simulink model "f28377S_DCDC_Buck"  (R2021b)
settings: Solver=FixedStepDiscrete  StartTime=0.0  StopTime=Inf  RelTol=1e-3  EnableMultiTasking=on
undefined symbols (not defined in the file or in its folder): GPTRIP1SEL, GPTRIP2SEL, TZ1, TZ2
libraries: c2837xDlib x3, c2802xlib x3, simulink x3, tiiqmathlib x2, c280xlib x2, c2000lib x1, demo_controls x1
settings Model: ExtModeTrigDuration=8  ExtModeTrigDurationFloating=10  ExtModeTrigDirection=either  ExtModeTrigLevel=0.500000  Creator=The MathWorks, Inc.  LastModifiedBy=The MathWorks, Inc.
settings SolverCC: AlgebraicLoopSolver=TrustRegion
settings DataIOCC: LimitDataPoints=on  SaveFormat=Array  SaveOutput=off  SaveTime=off  ReturnWorkspaceOutputs=off
settings OptimizationCC: DefaultParameterBehavior=Inlined  DefaultUnderspecifiedDataType=single  UseSpecifiedMinMax=on  InlineInvariantSignals=on  OptimizeBlockIOStorage=off  BufferReuse=off  GlobalBufferReuse=off  StrengthReduction=on  ExpressionFolding=off  PassReuseOutputArgsAs=Individual arguments  LocalBlockOutputs=off  NoFixptDivByZeroProtection=on  EfficientFloat2IntCast=on  LifeSpan=1  MaxStackSize=512  OptimizeDataStoreBuffers=off  BusAssignmentInplaceUpdate=off  EfficientTunableParamExpr=on
settings DebuggingCC: SolverPrmCheckMsg=warning  InheritedTsInSrcMsg=none  ParameterPrecisionLossMsg=none  SFUnexpectedBacktrackingDiag=warning  SFNoUnconditionalDefaultTransitionDiag=warning  SFExecutionAtInitializationDiag=none  SFMachineParentedDataDiag=warning  ArithmeticOperatorsInVariantConditions=warning
settings HardwareCC: ProdBitPerChar=16  ProdBitPerInt=16  ProdBitPerPointer=32  ProdBitPerSizeT=32  ProdBitPerPtrDiffT=32  ProdLargestAtomicInteger=Integer  ProdLargestAtomicFloat=None  ProdWordSize=16  ProdLongLongMode=on  ProdHWDeviceType=Texas Instruments->C2000
settings ModelReferenceCC: PropagateSignalLabelsOutOfModel=off
settings SFSimCC: SimUseLocalCustomCode=off  MATLABDynamicMemAlloc=off  CustomCodeUndefinedFunction=UseInterfaceOnly
settings RTWCC: Description=Embedded Coder  SystemTargetFile=ert.tlc  HardwareBoard=TI Delfino F2837xS  TemplateMakefile=ert_default_tmf  GenerateReport=on  RTWUseLocalCustomCode=off  Toolchain=Texas Instruments Code Composer Studio (C2000)  BuildConfiguration=Faster Runs  IncludeHyperlinkInReport=on  GenerateTraceInfo=on  GenerateTraceReport=on  GenerateTraceReportSl=on  GenerateTraceReportSf=on  GenerateTraceReportEml=on  GenerateCodeMetricsReport=on  GenerateCodeReplacementReport=on
settings CodeAppCC: IgnoreCustomStorageClasses=off  StateflowObjectComments=on
settings ERTTargetCC: CodeReplacementLibrary=TI C28x  UtilityFuncGeneration=Shared location  MultiwordLength=2048  IncludeMdlTerminateFcn=off  CombineSignalStateStructs=on  SupportAbsoluteTime=off  SupportNonFinite=off  SupportComplex=off  ExtModeMexFile=TIC2000ExternalModeOpen  ExtModeMexArgs=1 65 115385 30  ExtModeIntrfLevel=Level2 - Open  ERTFilePackagingFormat=Compact
settings ConfigComp: CovMetricSettings=dw  CovSaveCumulativeToWorkspaceVar=on  CovSaveSingleToWorkspaceVar=on  CovExternalEMLEnable=off  CovSFcnEnable=off
settings SimscapeCC: SimscapeNormalizeSystem=off
settings ConfigurationSet: Description=SimMechanics 2G

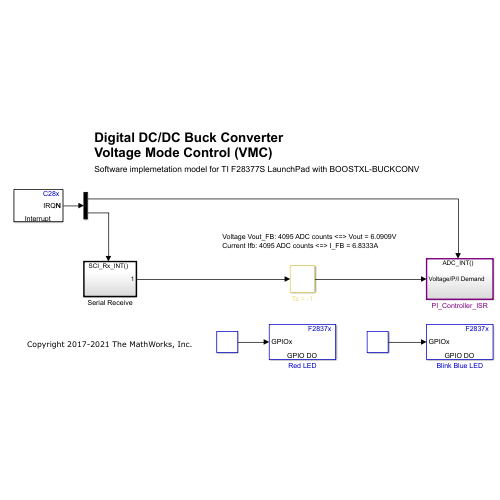
[thumbnail: Simulink's stored preview of the top-level diagram]
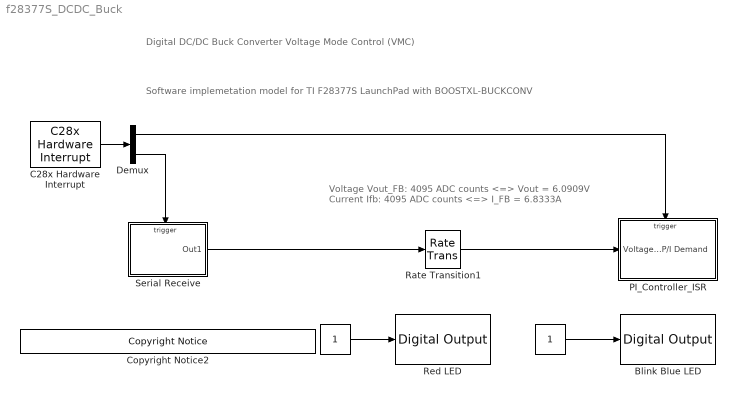
== system f28377S_DCDC_Buck ==
  note: Voltage Vout_FB: 4095 ADC counts <=> Vout = 6.0909V
      | Current Ifb: 4095 ADC counts <=> I_FB = 6.8333A
  note: Software implemetation model for TI F28377S LaunchPad with BOOSTXL-BUCKCONV
  note: Digital DC/DC Buck Converter
      | Voltage Mode Control (VMC)
  " " : Constant  OutDataTypeStr=uint16  SampleTime=0.5
  "   " : Constant  OutDataTypeStr=uint16  SampleTime=0.5
  Blink Blue LED : c2837xDlib/Digital Output  GPIO_Number=GPIO8~GPIO15  GPIO_Bit0=off  GPIO_BIT0_Toggle=off  GPIO_Bit1=off  GPIO_BIT1_Toggle=off  GPIO_Bit2=off  GPIO_BIT2_Toggle=off  GPIO_Bit3=off  GPIO_BIT3_Toggle=off  GPIO_Bit4=off  GPIO_BIT4_Toggle=on  GPIO_Bit5=on  GPIO_BIT5_Toggle=on  GPIO_Bit6=off  GPIO_BIT6_Toggle=off  GPIO_Bit7=off  GPIO_BIT7_Toggle=off
      settings: SourceProductBaseCode=TIC2000
  C28x Hardware Interrupt : c2000lib/Scheduling/C28x Hardware Interrupt  irqnumbers=[1 9]  pienumbers=[1 1]  irqpriorities=[30 50]  irqpreempts=[0 1]  showinput=off  dspchiptype=C280X
      settings: SourceProductBaseCode=TIC2000
  Copyright Notice2 : demo_controls/Copyright Notice  year=2017  prod=tic2000
      settings: SourceProductBaseCode=ME
  Demux : Demux  Outputs=2
  PI_Controller_ISR : Subsystem
  Rate Transition1 : RateTransition  Integrity=off
      settings: AttributesFormatString=Ts = %<OutPortSampleTime>
  Red LED : c2837xDlib/Digital Output  GPIO_Number=GPIO8~GPIO15  GPIO_Bit0=off  GPIO_BIT0_Toggle=off  GPIO_Bit1=off  GPIO_BIT1_Toggle=off  GPIO_Bit2=off  GPIO_BIT2_Toggle=off  GPIO_Bit3=off  GPIO_BIT3_Toggle=off  GPIO_Bit4=on  GPIO_BIT4_Toggle=off  GPIO_Bit5=off  GPIO_BIT5_Toggle=on  GPIO_Bit6=off  GPIO_BIT6_Toggle=off  GPIO_Bit7=off  GPIO_BIT7_Toggle=off
      settings: SourceProductBaseCode=TIC2000
  Serial Receive : Subsystem  SystemSampleTime=1e-3
  wires:
  Serial Receive/1(Out1) -> Rate Transition1/1
  " "/1 -> Blink Blue LED/1
  Demux/1 -> PI_Controller_ISR/Trigger
  Demux/2 -> Serial Receive/Trigger
  C28x Hardware Interrupt/1 -> Demux/1
  Rate Transition1/1 -> PI_Controller_ISR/1(Voltage/P/I Demand)
  "   "/1 -> Red LED/1

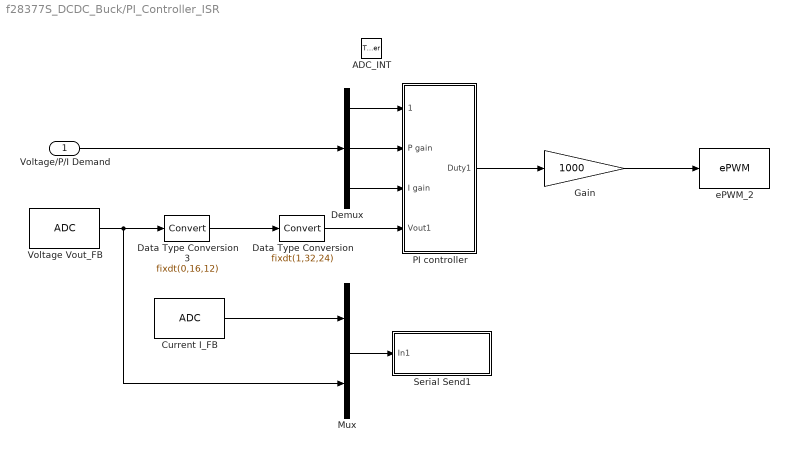
== system f28377S_DCDC_Buck/PI_Controller_ISR ==
  Voltage/P/I Demand : Inport
  ADC_INT : TriggerPort  TriggerType=function-call  VariantControl=Variant  PortDimensions=1
  Current I_FB : c2802xlib/ADC  blkParamProc=C2000_Type4  ADCModule=A  samplingMode=Single sample mode  ADCResolution=12-bit (Single-ended input)  useSOC1=SOC1  useSOC2=SOC0_SOC1  SOCAcquisitionWindow=14  SOCTriggerSource=ePWM2_ADCSOCA  SOCInterruptTrigger=No ADCINT  Ts=-1  dType=uint16  postInterrupt=off  interruptSel=ADCINT1  ADCINTContinuous=on  endma=off  chdma=1  conv1=ADCINA0  conv2=ADCINA0 and ADCINB0  conv1_Type4=ADCIN2  conv2_Type4=ADCIN0 and ADCIN1
  Data Type Conversion : DataTypeConversion  OutDataTypeStr=fixdt(1,32,24)  RndMeth=Simplest
      settings: AttributesFormatString=DataType = %<OutDataTypeStr>
  Data Type Conversion3 : DataTypeConversion  OutDataTypeStr=fixdt(0,16,12)  ConvertRealWorld=Stored Integer (SI)  RndMeth=Simplest
      settings: AttributesFormatString=DataType = %<OutDataTypeStr>
  Demux : Demux  Outputs=3
  Gain : Gain  Gain=1000  ParamDataTypeStr=int16  OutDataTypeStr=fixdt(1,32,20)  RndMeth=Simplest
  Mux : Mux  Inputs=2
  PI controller : Subsystem
  Serial Send1 : Subsystem
  Voltage Vout_FB : c2802xlib/ADC  blkParamProc=C2000_Type4  ADCModule=A  samplingMode=Single sample mode  ADCResolution=12-bit (Single-ended input)  useSOC1=SOC0  useSOC2=SOC0_SOC1  SOCAcquisitionWindow=14  SOCTriggerSource=ePWM2_ADCSOCA  SOCInterruptTrigger=No ADCINT  Ts=-1  dType=uint16  postInterrupt=on  interruptSel=ADCINT1  ADCINTContinuous=on  endma=off  chdma=1  conv1=ADCINA0  conv2=ADCINA0 and ADCINB0  conv1_Type4=ADCIN3  conv2_Type4=ADCIN0 and ADCIN1
  ePWM_2 : c2802xlib/ePWM  PwmType=C2000_Type4  useModule=ePWM2  ePWMxLINKTBPRD=Not Linked  periodUnits=Clock cycles  timerSource=Specify via dialog  timerPeriod_clk=1000  timerPeriod_sec=0.0001  tbshadow=Counter equals to zero  countingMode=Up  phaseActiveEnable=Disable  phaseDirection=Count down after sync  phaseActive=0  synchronizationEnable=off  dcaevt1Sync=off  dcbevt1Sync=off  synchronizationOption=Disable  perSynchronizationOption=Counter equals to period (CTR=PRD)  clockPrescale=1  HSclockPrescale=1  enswap=off  ePWMxAStatus=on  ePWMxAactionLogic1=Set  ePWMxAactionLogic2=Do nothing  ePWMxAactionLogic3=Clear  ePWMxAactionLogic4=Set  ePWMxAactionLogic5=Do nothing  ePWMxAactionLogic6=Do nothing  ePWMxACSFenable=off  ePWMxACSFvalue=Forcing disable  ePWMxASFreload=Zero  ePWMxBStatus=off  ePWMxBactionLogic1=Set  ePWMxBactionLogic2=Clear  ePWMxBactionLogic3=Do nothing  ePWMxBactionLogic4=Do nothing  ePWMxBactionLogic5=Clear  ePWMxBactionLogic6=Set  ePWMxBCSFenable=off  ePWMxBCSFvalue=Forcing disable  ePWMxBSFreload=Zero  ePWNxBOutWay=off  ePWMxLINKCMPA=Not Linked  CMPAUnits=Clock cycles  CMPASource=Input port  CMPAValue_per=50  CMPAValue_clk=0  enCMPAshadow=Counter equals to period (CTR=PRD)  ePWMxLINKCMPB=Not Linked  CMPBUnits=Clock cycles  CMPBSource=Specify via dialog  CMPBValue_per=50  CMPBValue_clk=1000-((15+54)*2)  enCMPBshadow=Counter equals to zero (CTR=Zero)  ePWMxLINKCMPC=Not Linked  CMPCUnits=Clock cycles  CMPCSource=Specify via dialog  CMPCValue_per=50  CMPCValue_clk=32000  enCMPCshadow=Counter equals to zero (CTR=Zero)  ePWMxLINKCMPD=Not Linked  CMPDUnits=Clock cycles  CMPDSource=Specify via dialog  CMPDValue_per=50  CMPDValue_clk=32000  enCMPDshadow=Counter equals to zero (CTR=Zero)  enableDBePWMxA=on  enableDBePWMxB=on  enhalfcycle=off  DBpolarity=Active high complementary (AHC)  DBedgeDelay=Positive  DBSource_ePWMxA=ePWMxA  DBSource_ePWMxB=ePWMxA  DBPeriodUnits=Clock cycles  DBperiodSource=Specify via dialog  REDperiod=20  FEDperiod=20  REDperiod_sec=0  FEDperiod_sec=0  LoadModeDBRED=Immediate without using shadow  LoadModeDBFED=Immediate without using shadow  adcstartModuleA=on  adcrequestEventA=First event  adcstartEventA=Digital Compare Module A Event 1 start of conversion (DCAEVT1.soc)  adcstartEventA_type2=Counter is incrementing and equals to the compare B register (CTRU=CMPB)  adcstartModuleB=off  adcrequestEventB=First event  adcstartEventB=Counter equals to zero (CTR=Zero)  adcstartEventB_type2=Counter equals to zero (CTR=Zero)  intEn=off  intPrd=First event  intSel=Counter equals to zero (CTR=Zero)  intSel_type2=Counter equals to zero (CTR=Zero)  hrpe=off  enHRPWM=off  HRPWM_LoadMode=Counter equals to period (CTR=PRD)  HRPWM_CTLMode=Duty or Period control mode  HRPWM_EDGMode=Both edge  hrpeb=off  enHRPWMB=off  HRPWM_LoadModeB=Counter equals to zero (CTR=ZERO)  HRPWM_CTLModeB=Duty or Period control mode  HRPWM_EDGModeB=Both edge  enHRDBRED=off  enHRDBFED=off  enSFO=on  enautoconv=on  chopperEnable=off  chopperFrequency=1  chopperFirstwidth=1  chopperDuty=12.5%  tripZonesource=Specify via dialog  tzselOSHT1=off  tzselOSHT2=off  tzselOSHT3=off  tzselOSHDCAEV1=off  tzselOSHDCBEV1=off  tzselCBC1=off  tzselCBC2=off  tzselCBC3=off  tzselCBCDCAEV2=off  tzselCBCDCBEV2=off  tzselOSHT4=off  tzselOSHT5=off  tzselOSHT6=off  tzselCBC4=off  tzselCBC5=off  tzselCBC6=off  enTzOstIntr=off  enTzCbcIntr=off  enTzDCAEVT1Intr=off  enTzDCAEVT2Intr=off  enTzDCBEVT1Intr=off  enTzDCBEVT2Intr=off  ePWMxAforced=No action  ePWMxBforced=No action  DCAEVT1forced=No action  DCBEVT1forced=No action  DCAEVT2forced=No action  DCBEVT2forced=No action  dcah=Trip Zone 1 input (TZ1)  dcal=Trip Zone 2 input (TZ2)  dcbh=Trip Zone 1 input (TZ1)  dcbl=Trip Zone 2 input (TZ2)  dcah_type2=GPTRIP1SEL/(TZ1)  dcal_type2=GPTRIP2SEL/(TZ2)  dcbh_type2=GPTRIP1SEL/(TZ1)  dcbl_type2=GPTRIP2SEL/(TZ2)  gendcaevt1=Event disabled  gendcaevt2=Event disabled  gendcbevt1=Event disabled  gendcbevt2=Event disabled  dcaevt1src=DCAEVT1 with sync  dcaevt2src=DCAEVT2 with sync  dcbevt1src=DCBEVT1 with sync  dcbevt2src=DCBEVT2 with sync  pulsesel=Counter equals to zero (CTR=Zero)  blankinv=off  blankoffset=0  blankwidth=0  evsrcsel=Filtered version of DCAEVT1 (DCAEVT1FILT)  encape=off
  wires:
  Data Type Conversion3/1 -> Data Type Conversion/1
  Gain/1 -> ePWM_2/1
  PI controller/1(Duty1) -> Gain/1
  Data Type Conversion/1 -> PI controller/4(Vout1)
  Mux/1 -> Serial Send1/1(In1)
  Demux/1 -> PI controller/1(Vout1Ref)
  Demux/2 -> PI controller/2(P gain)
  Demux/3 -> PI controller/3(I gain)
  Voltage/P/I Demand/1 -> Demux/1
  Current I_FB/1 -> Mux/1
  Voltage Vout_FB/1 -> Mux/2, Data Type Conversion3/1

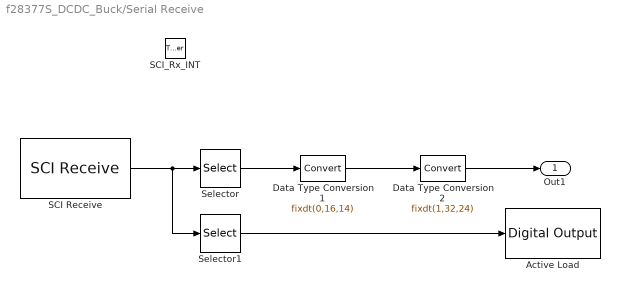
== system f28377S_DCDC_Buck/Serial Receive ==
  SCI_Rx_INT : TriggerPort  TriggerType=function-call  VariantControl=Variant
  Active Load : c2837xDlib/Digital Output  GPIO_Number=GPIO16~GPIO23  GPIO_Bit0=off  GPIO_BIT0_Toggle=off  GPIO_Bit1=off  GPIO_BIT1_Toggle=off  GPIO_Bit2=on  GPIO_BIT2_Toggle=off  GPIO_Bit3=off  GPIO_BIT3_Toggle=off  GPIO_Bit4=off  GPIO_BIT4_Toggle=on  GPIO_Bit5=off  GPIO_BIT5_Toggle=off  GPIO_Bit6=off  GPIO_BIT6_Toggle=off  GPIO_Bit7=off  GPIO_BIT7_Toggle=off
      settings: SourceProductBaseCode=TIC2000
  Data Type Conversion1 : DataTypeConversion  OutDataTypeStr=fixdt(0,16,14)  ConvertRealWorld=Stored Integer (SI)  RndMeth=Simplest
      settings: AttributesFormatString=DataType = %<OutDataTypeStr>
  Data Type Conversion2 : DataTypeConversion  OutDataTypeStr=fixdt(1,32,24)  RndMeth=Simplest
      settings: AttributesFormatString=DataType = %<OutDataTypeStr>
  SCI Receive : c280xlib/SCI Receive  sciModule=A  dataHead='S'  dataTail='E'  dataType=uint16  dataDim=4  initValue=0  errOption=Output the last received value  errValue=0  sampleTime=-1  outputStatus=off  postInterrupt=on  numFifo=10
      settings: SourceProductBaseCode=TIC2000
  Selector : Selector  InputPortWidth=4  IndexOptions=Index vector (dialog)  Indices=[1 2 3]  OutputSizes=1
  Selector1 : Selector  InputPortWidth=4  IndexOptions=Index vector (dialog)  Indices=4  OutputSizes=1
  Out1 : Outport  InitialOutput=[0 0.002 0.003]  VectorParamsAs1DForOutWhenUnconnected=off
  wires:
  SCI Receive/1 -> Selector1/1, Selector/1
  Selector/1 -> Data Type Conversion1/1
  Selector1/1 -> Active Load/1
  Data Type Conversion1/1 -> Data Type Conversion2/1
  Data Type Conversion2/1 -> Out1/1

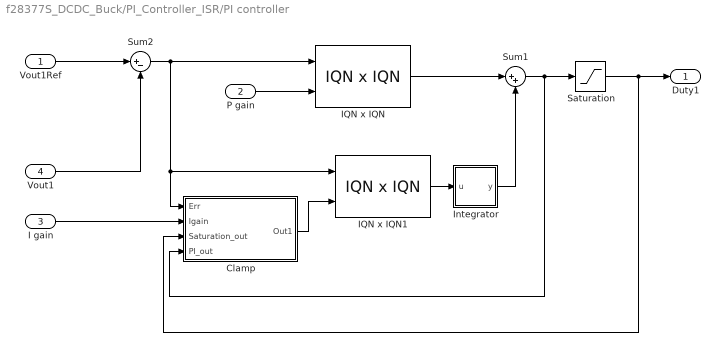
== system f28377S_DCDC_Buck/PI_Controller_ISR/PI controller ==
  Vout1Ref : Inport
  P gain : Inport  Port=2
  I gain : Inport  Port=3
  Vout1 : Inport  Port=4
  Clamp : Subsystem
  IQN x IQN : tiiqmathlib/IQN x IQN  multiplyOption=Multiply
      settings: SourceProductBaseCode=TIC2000
  IQN x IQN1 : tiiqmathlib/IQN x IQN  multiplyOption=Multiply
      settings: SourceProductBaseCode=TIC2000
  Integrator : Subsystem
  Saturation : Saturate  UpperLimit=0.6  LowerLimit=0  RndMeth=Simplest
      settings: AttributesFormatString=|
      | ULim = %<UpperLimit>
      | LLim = %<LowerLimit>
  Sum1 : Sum  Inputs=|++  RndMeth=Simplest  OutDataTypeStr=Inherit: Same as first input
  Sum2 : Sum  Inputs=|+-  RndMeth=Simplest  OutDataTypeStr=Inherit: Same as first input
  Duty1 : Outport  VectorParamsAs1DForOutWhenUnconnected=off
  wires:
  P gain/1 -> IQN x IQN/2
  Vout1Ref/1 -> Sum2/1
  Integrator/1(y) -> Sum1/2
  Vout1/1 -> Sum2/2
  Sum2/1 -> IQN x IQN/1, IQN x IQN1/1, Clamp/1(Err)
  Sum1/1 -> Clamp/4(PI_out), Saturation/1
  Saturation/1 -> Clamp/3(Saturation_out), Duty1/1
  IQN x IQN/1 -> Sum1/1
  IQN x IQN1/1 -> Integrator/1(u)
  I gain/1 -> Clamp/2(Igain)
  Clamp/1(Out1) -> IQN x IQN1/2

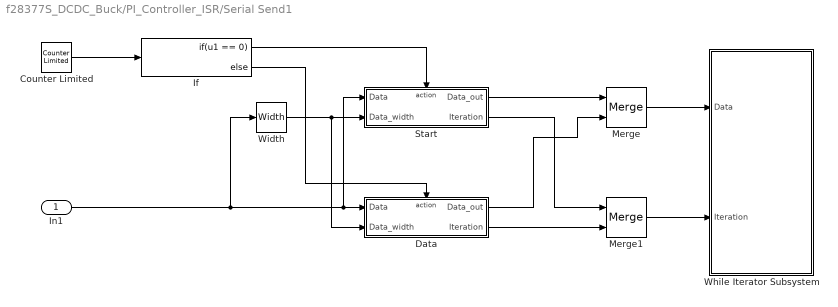
== system f28377S_DCDC_Buck/PI_Controller_ISR/Serial Send1 ==
  In1 : Inport
  Counter Limited : simulink/Sources/Counter Limited  uplimit=11999  tsamp=-1
  Data : Subsystem  TreatAsAtomicUnit=on
  If : If  IfExpression=u1 == 0
  Merge : Merge
  Merge1 : Merge
  Start : Subsystem  TreatAsAtomicUnit=on
  While Iterator Subsystem : Subsystem  TreatAsAtomicUnit=on
  Width : Width  OutDataTypeMode=All ports same datatype  DataType=uint16
  wires:
  If/1 -> Start/Action
  If/2 -> Data/Action
  Counter Limited/1 -> If/1
  Start/1(Data_out) -> Merge/1
  Data/1(Data_out) -> Merge/2
  Merge/1 -> While Iterator Subsystem/1(Data)
  Merge1/1 -> While Iterator Subsystem/2(Iteration)
  Start/2(Iteration) -> Merge1/1
  Data/2(Iteration) -> Merge1/2
  Width/1 -> Data/2(Data_width), Start/2(Data_width)
  In1/1 -> Width/1, Start/1(Data), Data/1(Data)

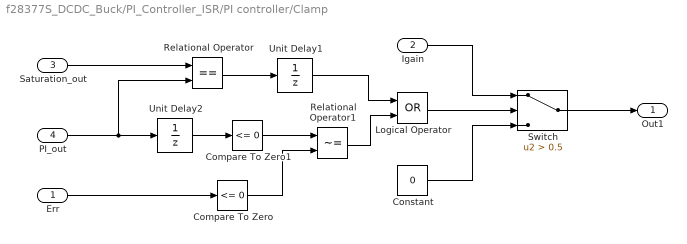
== system f28377S_DCDC_Buck/PI_Controller_ISR/PI controller/Clamp ==
  Err : Inport
  Igain : Inport  Port=2
  Saturation_out : Inport  Port=3
  PI_out : Inport  Port=4
  Compare To Zero : simulink/Logic and Bit Operations/Compare To Zero  relop=<=  OutDataTypeStr=boolean
  Compare To Zero1 : simulink/Logic and Bit Operations/Compare To Zero  relop=<=  OutDataTypeStr=boolean
  Constant : Constant  Value=0  OutDataTypeStr=fixdt(1,32,24)  SampleTime=-1
  Logical Operator : Logic  Operator=OR  AllPortsSameDT=off  OutDataTypeStr=boolean
  Relational Operator : RelationalOperator  Operator===  OutDataTypeStr=boolean  RndMeth=Nearest
  Relational Operator1 : RelationalOperator  Operator=~=  OutDataTypeStr=boolean  RndMeth=Nearest
  Switch : Switch  Criteria=u2 > Threshold  Threshold=0.5
  Unit Delay1 : UnitDelay  SampleTime=-1  HasFrameUpgradeWarning=on
  Unit Delay2 : UnitDelay  SampleTime=-1  HasFrameUpgradeWarning=on
  Out1 : Outport  VectorParamsAs1DForOutWhenUnconnected=off
  wires:
  Relational Operator1/1 -> Logical Operator/2
  Relational Operator/1 -> Unit Delay1/1
  Compare To Zero/1 -> Relational Operator1/2
  PI_out/1 -> Relational Operator/2, Unit Delay2/1
  Unit Delay2/1 -> Compare To Zero1/1
  Compare To Zero1/1 -> Relational Operator1/1
  Unit Delay1/1 -> Logical Operator/1
  Constant/1 -> Switch/3
  Logical Operator/1 -> Switch/2
  Switch/1 -> Out1/1
  Err/1 -> Compare To Zero/1
  Saturation_out/1 -> Relational Operator/1
  Igain/1 -> Switch/1

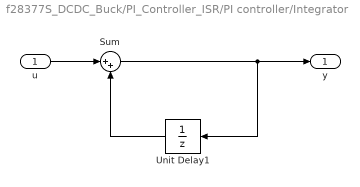
== system f28377S_DCDC_Buck/PI_Controller_ISR/PI controller/Integrator ==
  u : Inport
  Sum : Sum  Inputs=|++  RndMeth=Simplest  OutDataTypeStr=Inherit: Same as first input
  Unit Delay1 : UnitDelay  SampleTime=-1  HasFrameUpgradeWarning=on
  y : Outport  VectorParamsAs1DForOutWhenUnconnected=off
  wires:
  Sum/1 -> Unit Delay1/1, y/1
  Unit Delay1/1 -> Sum/2
  u/1 -> Sum/1

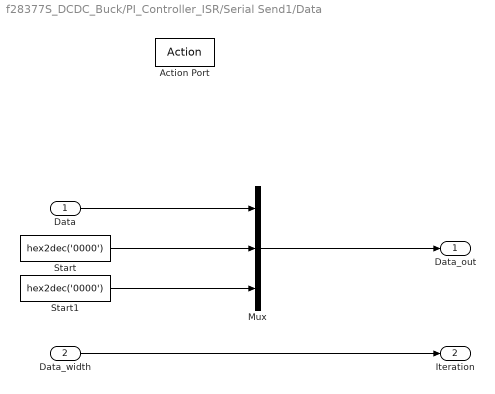
== system f28377S_DCDC_Buck/PI_Controller_ISR/Serial Send1/Data ==
  Data : Inport
  Data_width : Inport  Port=2
  Action Port : ActionPort  ActionPortLabel=else { }
  Mux : Mux  Inputs=3
  Start : Constant  Value=hex2dec('0000')  OutDataTypeStr=uint16
  Start1 : Constant  Value=hex2dec('0000')  OutDataTypeStr=uint16
  Data_out : Outport  VectorParamsAs1DForOutWhenUnconnected=off
  Iteration : Outport  Port=2  VectorParamsAs1DForOutWhenUnconnected=off
  wires:
  Start/1 -> Mux/2
  Mux/1 -> Data_out/1
  Data/1 -> Mux/1
  Data_width/1 -> Iteration/1
  Start1/1 -> Mux/3

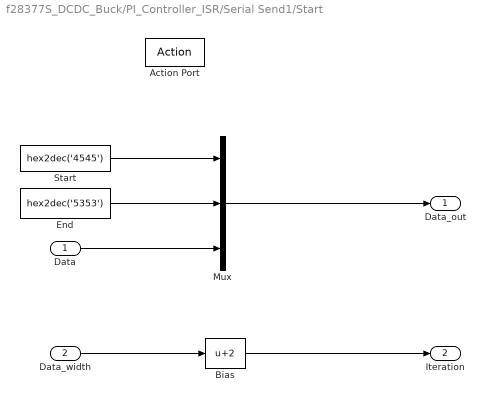
== system f28377S_DCDC_Buck/PI_Controller_ISR/Serial Send1/Start ==
  Data : Inport
  Data_width : Inport  Port=2
  Action Port : ActionPort  ActionPortLabel=if { }
  Bias : Bias  Bias=2
  End : Constant  Value=hex2dec('5353')  OutDataTypeStr=uint16
  Mux : Mux  Inputs=3
  Start : Constant  Value=hex2dec('4545')  OutDataTypeStr=uint16
  Data_out : Outport  VectorParamsAs1DForOutWhenUnconnected=off
  Iteration : Outport  Port=2  VectorParamsAs1DForOutWhenUnconnected=off
  wires:
  End/1 -> Mux/2
  Mux/1 -> Data_out/1
  Data_width/1 -> Bias/1
  Bias/1 -> Iteration/1
  Data/1 -> Mux/3
  Start/1 -> Mux/1

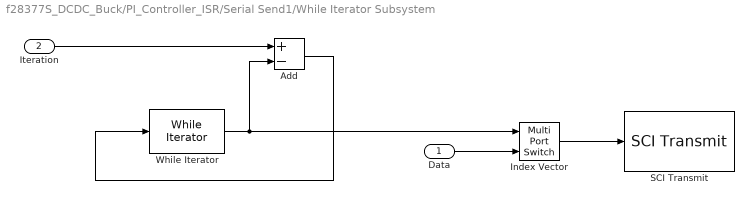
== system f28377S_DCDC_Buck/PI_Controller_ISR/Serial Send1/While Iterator Subsystem ==
  Data : Inport
  Iteration : Inport  Port=2
  Add : Sum  Inputs=+-  OutDataTypeStr=Inherit: Same as first input
  Index Vector : MultiPortSwitch  Inputs=1
  SCI Transmit : c280xlib/SCI Transmit  sciModule=A  dataHead=''  dataTail=''  postInterrupt=off  numFifo=1
  While Iterator : WhileIterator  MaxIters=-1  WhileBlockType=do-while  ShowIterationPort=on  OutputDataType=int16
  wires:
  Iteration/1 -> Add/1
  Add/1 -> While Iterator/1
  Index Vector/1 -> SCI Transmit/1
  Data/1 -> Index Vector/2
  While Iterator/1 -> Index Vector/1, Add/2
